simulink model "MSDR_v1.1"  (R2018a)
settings: Solver=ode3  StartTime=0.0  StopTime=21600  FixedStep=0.05
values from neighbouring files (symbols this model uses):
  a_f = -3.22E-5    (= -3.22e-05)    [MSDR_parameters.m]
  a_g = +2.35E-5    (= 2.35e-05)    [MSDR_parameters.m]
  A_s = 1.2245    [MSDR_parameters.m]
  beta = [0.000223, 0.001457, 0.001307, 0.002628, 0.000766, 0.000280]    [MSDR_parameters.m]
  beta_t = sum(beta)    [MSDR_parameters.m]
  ce1 = 1.2471e-07    [MSDR_parameters.m]
  ce2 = 5.3816e-14    [MSDR_parameters.m]
  ce3 = 3.3721e-08    [MSDR_parameters.m]
  Cp_fw = 3200.448e-6    (= 0.003200448)    [MSDR_parameters.m]
  Cp_hr = 0.0021520    (= 0.002152)    [MSDR_parameters.m]
  Cp_p = Cp_s_shx    (= 0.00154912)    [MSDR_parameters.m]
  Cp_s = Cp_s*1e-6    (= 3.588208e-09)    [MSDR_parameters.m]
  Cp_s_shx = 1549.12e-6    (= 0.00154912)    [MSDR_parameters.m]
  Cp_sc = 4761.392e-6    (= 0.004761392)    [MSDR_parameters.m]
  Cp_w = 456.056e-6    (= 0.000456056)    [MSDR_parameters.m]
  D_it = 0.0141478    [MSDR_parameters.m]
  D_ot = 0.015875    [MSDR_parameters.m]
  dHs_dPs = -0.042433622114357    (= -0.0424336221144)    [MSDR_parameters.m]
  eta_hp_isen = 0.861    [MSDR_parameters.m]
  eta_lp_isen = 0.861    [MSDR_parameters.m]
  gamma_I = 5.1135e-2    (= 0.051135)    [MSDR_parameters.m]
  gamma_Xe = 1.1628e-2    (= 0.011628)    [MSDR_parameters.m]
  H_fwh1 = 0.46009    [MSDR_parameters.m]
  h_fwh1 = 0.5927    [MSDR_parameters.m]
  H_fwh2 = 0.6784    [MSDR_parameters.m]
  h_fwh2 = 0.5927    [MSDR_parameters.m]
  H_lp_isen = 958.4*1054.35e-6/0.45359237    (= 2.22774699671)    [MSDR_parameters.m]
  H_nc = 3.2952    [MSDR_parameters.m]
  h_pw = h_s_shx    (= 0.00567446)    [MSDR_parameters.m]
  H_rh = 2.8115    [MSDR_parameters.m]
  h_wb = 13349.334646671E-6    (= 0.0133493346467)    [MSDR_parameters.m]
  h_ws = 5732.378387768E-6    (= 0.00573237838777)    [MSDR_parameters.m]
  h_wsc = 8385.005556375E-6    (= 0.00838500555638)    [MSDR_parameters.m]
  hA_fg = [h_fg*A_fg/2, h_fg*A_fg/2]    [MSDR_parameters.m]
  hA_p_phx1 = h_p_phx*A_p_phx    [MSDR_parameters.m]
  hA_p_phx2 = h_p_phx*A_p_phx    [MSDR_parameters.m]
  hA_p_phx3 = h_p_phx*A_p_phx    [MSDR_parameters.m]
  hA_p_phx4 = h_p_phx*A_p_phx    [MSDR_parameters.m]
  hA_p_phx5 = h_p_phx*A_p_phx    [MSDR_parameters.m]
  hA_p_phx6 = h_p_phx*A_p_phx    [MSDR_parameters.m]
  hA_p_shx1 = h_p_shx*A_p_shx    [MSDR_parameters.m]
  hA_p_shx2 = h_p_shx*A_p_shx    [MSDR_parameters.m]
  hA_p_shx3 = h_p_shx*A_p_shx    [MSDR_parameters.m]
  hA_p_shx4 = h_p_shx*A_p_shx    [MSDR_parameters.m]
  hA_p_shx5 = h_p_shx*A_p_shx    [MSDR_parameters.m]
  hA_p_shx6 = h_p_shx*A_p_shx    [MSDR_parameters.m]
  hA_s_phx1 = h_s_phx*A_s_phx    [MSDR_parameters.m]
  hA_s_phx2 = h_s_phx*A_s_phx    [MSDR_parameters.m]
  hA_s_phx3 = h_s_phx*A_s_phx    [MSDR_parameters.m]
  hA_s_phx4 = h_s_phx*A_s_phx    [MSDR_parameters.m]
  hA_s_phx5 = h_s_phx*A_s_phx    [MSDR_parameters.m]
  hA_s_phx6 = h_s_phx*A_s_phx    [MSDR_parameters.m]
  hA_s_shx1 = h_s_shx*A_s_shx    [MSDR_parameters.m]
  hA_s_shx2 = h_s_shx*A_s_shx    [MSDR_parameters.m]
  hA_s_shx3 = h_s_shx*A_s_shx    [MSDR_parameters.m]
  hA_s_shx4 = h_s_shx*A_s_shx    [MSDR_parameters.m]
  hA_s_shx5 = h_s_shx*A_s_shx    [MSDR_parameters.m]
  hA_s_shx6 = h_s_shx*A_s_shx    [MSDR_parameters.m]
  I_0 = gamma_I*Sig_f_msdr*phi_0/lam_I    (= 4.38204721773e+16)    [MSDR_parameters.m]
  Ifa = [0.25, 0.25]    [MSDR_parameters.m]
  Ifb = [0.25, 0.25]    [MSDR_parameters.m]
  Ig = [0.5, 0.5]    [MSDR_parameters.m]
  K_1 = 11.632248097704855    (= 11.6322480977)    [MSDR_parameters.m]
  K_4 = b(1)    [MSDR_parameters.m]
  K_5 = a(1)    [MSDR_parameters.m]
  K_b = 12.834854076292217    (= 12.8348540763)    [MSDR_parameters.m]
  K_b_hp = 0.1634    [MSDR_parameters.m]
  K_b_lp = 0.2174    [MSDR_parameters.m]
  K_sc = -17.615718797133468    (= -17.6157187971)    [MSDR_parameters.m]
  ka = [0.235, 0.235]    [MSDR_parameters.m]
  kb = [0.235, 0.235]    [MSDR_parameters.m]
  kga = [0.015, 0.015]    [MSDR_parameters.m]
  kgb = [0.015, 0.015]    [MSDR_parameters.m]
  L = 8.5344    [MSDR_parameters.m]
  L_b = 2.3645    [MSDR_parameters.m]
  L_s = 4.723    [MSDR_parameters.m]
  Lam = 2.400E-04    (= 0.00024)    [MSDR_parameters.m]
  lam = [0.0124, 0.0305, 0.111, 0.301, 1.14, 3.01]    [MSDR_parameters.m]
  lam_bubl = 2.0e-2    (= 0.02)    [MSDR_parameters.m]
  lam_I = 2.875e-5    (= 2.875e-05)    [MSDR_parameters.m]
  lam_Xe = 2.0916e-5    (= 2.0916e-05)    [MSDR_parameters.m]
  m_3m = W_3*2    (= 8618.207327)    [MSDR_parameters.m]
  m_fm = W_f*2    (= 9978.96)    [MSDR_parameters.m]
  m_sb = 1717    [MSDR_parameters.m]
  M_stm = 0.018    [MSDR_parameters.m]
  mb_cpb = 2.689619410657651e+00    (= 2.68961941066)    [MSDR_parameters.m]
  mcp_fa = mfa*Cp_f    [MSDR_parameters.m]
  mcp_fb = mfb*Cp_f    [MSDR_parameters.m]
  mcp_g = mg*Cp_g    [MSDR_parameters.m]
  mcp_p_phx1 = Cp_p_phx*mp_phx1    [MSDR_parameters.m]
  mcp_p_phx2 = Cp_p_phx*mp_phx2    [MSDR_parameters.m]
  mcp_p_phx3 = Cp_p_phx*mp_phx3    [MSDR_parameters.m]
  mcp_p_phx4 = Cp_p_phx*mp_phx4    [MSDR_parameters.m]
  mcp_p_phx5 = Cp_p_phx*mp_phx5    [MSDR_parameters.m]
  mcp_p_phx6 = Cp_p_phx*mp_phx6    [MSDR_parameters.m]
  mcp_p_shx1 = Cp_p_shx*mp_shx1    [MSDR_parameters.m]
  mcp_p_shx2 = Cp_p_shx*mp_shx2    [MSDR_parameters.m]
  mcp_p_shx3 = Cp_p_shx*mp_shx3    [MSDR_parameters.m]
  mcp_p_shx4 = Cp_p_shx*mp_shx4    [MSDR_parameters.m]
  mcp_p_shx5 = Cp_p_shx*mp_shx5    [MSDR_parameters.m]
  mcp_p_shx6 = Cp_p_shx*mp_shx6    [MSDR_parameters.m]
  mcp_s_phx1 = Cp_s_phx*ms_phx1    [MSDR_parameters.m]
  mcp_s_phx2 = Cp_s_phx*ms_phx2    [MSDR_parameters.m]
  mcp_s_phx3 = Cp_s_phx*ms_phx3    [MSDR_parameters.m]
  mcp_s_phx4 = Cp_s_phx*ms_phx4    [MSDR_parameters.m]
  mcp_s_phx5 = Cp_s_phx*ms_phx5    [MSDR_parameters.m]
  mcp_s_phx6 = Cp_s_phx*ms_phx6    [MSDR_parameters.m]
  mcp_s_shx1 = Cp_s_shx*ms_shx1    [MSDR_parameters.m]
  mcp_s_shx2 = Cp_s_shx*ms_shx1    [MSDR_parameters.m]
  mcp_s_shx3 = Cp_s_shx*ms_shx1    [MSDR_parameters.m]
  mcp_s_shx4 = Cp_s_shx*ms_shx1    [MSDR_parameters.m]
  mcp_s_shx5 = Cp_s_shx*ms_shx1    [MSDR_parameters.m]
  mcp_s_shx6 = Cp_s_shx*ms_shx1    [MSDR_parameters.m]
  mcp_t_phx1 = Cp_t_phx*mt_phx1    [MSDR_parameters.m]
  mcp_t_phx2 = Cp_t_phx*mt_phx2    [MSDR_parameters.m]
  mcp_t_phx3 = Cp_t_phx*mt_phx3    [MSDR_parameters.m]
  mcp_t_phx4 = Cp_t_phx*mt_phx4    [MSDR_parameters.m]
  mcp_t_phx5 = Cp_t_phx*mt_phx5    [MSDR_parameters.m]
  mcp_t_phx6 = Cp_t_phx*mt_phx6    [MSDR_parameters.m]
  mcp_t_shx1 = Cp_t_phx*mt_shx1    [MSDR_parameters.m]
  ... (+177 more)
undefined symbols (not defined in the file or in its folder): C0, H_rh_table, H_rh_table1, H_rh_table2, H_rhvap_table, H_s_table, H_table, hA_p_thx1, hA_p_thx2, hA_p_thx3, hA_s_thx1, hA_s_thx2, hA_s_thx3, mcp_p_thx1, mcp_p_thx2, mcp_p_thx3, mcp_s_thx1, mcp_s_thx2, mcp_s_thx3, mcp_t_thx1, mcp_t_thx2, mcp_t_thx3, mp_thx1, mp_thx2, mp_thx3, ms_thx1, ms_thx2, ms_thx3, P_nc_table, P_rh_table, P_rh_table1, pres_table, rho_rh_table, rho_table, SV_nc_table, T0_p_thx1, T0_p_thx2, T0_p_thx3, T0_s_thx1, T0_s_thx2, T0_s_thx3, T0_t_thx1, T0_t_thx2, T0_t_thx3, temp_table, u14, Wp_thx1, Wp_thx2
libraries: simulink x13
(part 3 of 6)

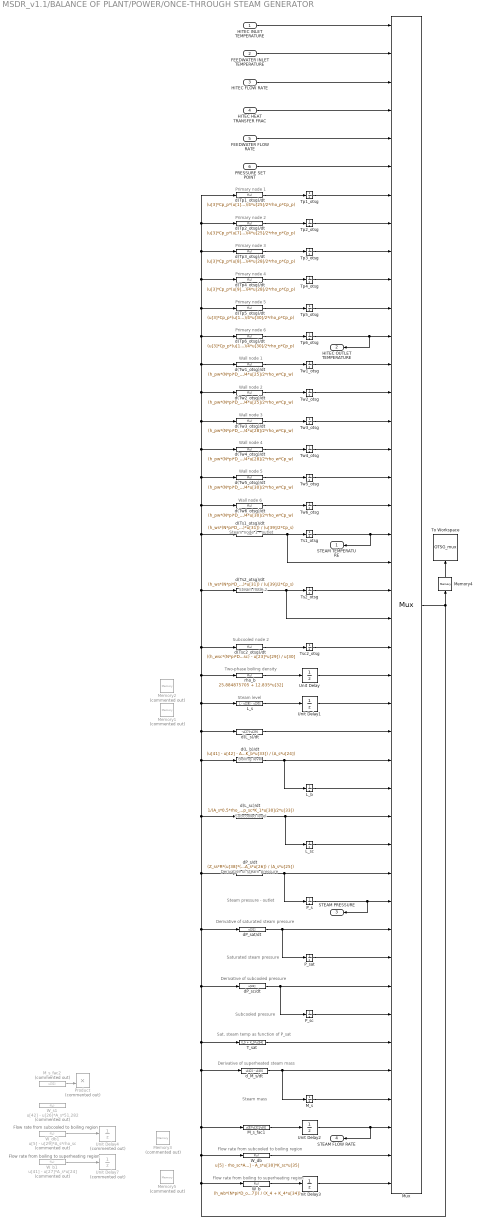
== system MSDR_v1.1/BALANCE OF PLANT/POWER/ONCE-THROUGH STEAM GENERATOR ==
  note: Primary node 1
  note: Primary node 2
  note: Primary node 3
  note: Primary node 4
  note: Primary node 5
  note: Primary node 6
  note: Wall node 1
  note: Wall node 2
  note: Wall node 3
  note: Wall node 4
  note: Wall node 5
  note: Wall node 6
  note: Steam node 1 - outlet
  note: Steam level
  note: Boiling level
  note: Subcooled level
  note: Derivative of saturated steam pressure
  note: Sat. steam temp as function of P_sat
  note: Saturated steam pressure
  note: Subcooled pressure
  note: Derivative of steam pressure
  note: Derivative of subcooled pressure
  note: Steam pressure - outlet
  note: Subcooled node 2
  note: Steam node 2
  note: Two-phase boiling density
  note: Derivative of superheated steam mass
  note: Steam mass
  note: Flow rate from subcooled to boiling region
  note: Flow rate from boiling to superheating region
  note: Flow rate from subcooled to boiling region
  note: Flow rate from boiling to superheating region
  HITEC INLET TEMPERATURE : Inport
  FEEDWATER INLET TEMPERATURE : Inport  Port=2
  HITEC FLOW RATE : Inport  Port=3
  HITEC HEAT TRANSFER FRAC : Inport  Port=4
  FEEDWATER FLOW RATE : Inport  Port=5
  PRESSURE SET POINT : Inport  Port=6
  L_b : Integrator  InitialCondition=L_b
  L_s : Fcn  Expr=L - u[28] - u[30]
  L_sc : Integrator  InitialCondition=.5344
  M_s : Integrator  InitialCondition=A_s*rho_s*L_s
  M_s_fac1 : Fcn  Expr=u[5]*u[32]/u[6]
  M_s_fac2 : Fcn  Commented=on  Expr=u[32]
  Memory1 : Memory  Commented=on  InitialCondition=L_s  InheritSampleTime=on
  Memory2 : Memory  Commented=on  InitialCondition=rho_b  InheritSampleTime=on
  Memory3 : Memory  Commented=on  InitialCondition=W_fw  InheritSampleTime=on
  Memory4 : Memory  InheritSampleTime=on
  Memory5 : Memory  Commented=on  InitialCondition=W_fw  InheritSampleTime=on
  Mux : Mux  Inputs=42
      settings: DisplayOption=signals
  P_s : Integrator  InitialCondition=P_s
  P_sat : Integrator  InitialCondition=P_sat
  P_sc : Integrator  InitialCondition=P_sc
  Product : Product  Commented=on
  T_sat : Fcn  Expr=X_5 + K_5*u[34]
  To Workspace : ToWorkspace  VariableName=OTSG_mux  SampleTime=-1
  Tp1_otsg : Integrator  InitialCondition=T_p1
  Tp2_otsg : Integrator  InitialCondition=T_p2
  Tp3_otsg : Integrator  InitialCondition=T_p3
  Tp4_otsg : Integrator  InitialCondition=T_p4
  Tp5_otsg : Integrator  InitialCondition=T_p5
  Tp6_otsg : Integrator  InitialCondition=T_p6
  Ts1_otsg : Integrator  InitialCondition=T_s1
  Ts2_otsg : Integrator  InitialCondition=T_s2
  Tsc2_otsg : Integrator  InitialCondition=T_sc2
  Tw1_otsg : Integrator  InitialCondition=T_w1
  Tw2_otsg : Integrator  InitialCondition=T_w2
  Tw3_otsg : Integrator  InitialCondition=T_w3
  Tw4_otsg : Integrator  InitialCondition=T_w4
  Tw5_otsg : Integrator  InitialCondition=T_w5
  Tw6_otsg : Integrator  InitialCondition=T_w6
  Unit Delay : UnitDelay  InitialCondition=rho_b  SampleTime=-1
  Unit Delay1 : UnitDelay  InitialCondition=L_s  SampleTime=-1
  Unit Delay2 : UnitDelay  InitialCondition=W_fw  SampleTime=-1
  Unit Delay3 : UnitDelay  InitialCondition=W_fw  SampleTime=-1
  Unit Delay4 : UnitDelay  Commented=on  InitialCondition=W_fw  SampleTime=-1
  Unit Delay7 : UnitDelay  Commented=on  InitialCondition=W_fw  SampleTime=-1
  W_b : Fcn  Expr=(h_wb*(N*pi*D_ot*u[28])*(0.5*u[15] + 0.5*u[16] - u[37])) / (X_4 + K_4*u[34])
  W_b1 : Fcn  Commented=on  Expr=u[41] - u[27]*A_s*u[24]
  W_db : Fcn  Expr=u[5] - rho_sc*A_s*u[29] - A_s*u[30]*K_sc*u[35]
  W_db1 : Fcn  Commented=on  Expr=u[5] - u[29]*A_s*rho_sc
  W_s1 : Fcn  Commented=on  Expr=u[42] - u[26]*A_s*51.282
  d(L_b)/dt : Fcn  Expr=(u[41] - u[42] - A_s*u[28]*K_b*u[33]) / (A_s*u[24])
  d(L_s)/dt : Fcn  Expr=-u[27]-u[29]
  d(L_sc)/dt : Fcn  Expr=1/(A_s*0.5*rho_sc*Cp_sc*(u[23] - u[37])) * (h_wsc*N*pi*D_ot*u[30]/2*(u[17] - u[37]) + u[5]*Cp_sc*(u[23] - u[37]) - A_s*u[30]/2*(K_sc*Cp_sc*(u[23] - 2*u[37]) - 1)*u[35] - A_s*rho_sc*Cp_sc*K_1*u[30]/2*u[33])
  d(Tp1_otsg)/dt : Fcn  Expr=(u[3]*Cp_p*(u[1] - u[7]) + h_pw*(N*pi*D_it*u[25]/2)*(u[13] - u[7])) / (N*pi*(D_it^2)/4*u[25]/2*rho_p*Cp_p)
  d(Tp2_otsg)/dt : Fcn  Expr=(u[3]*Cp_p*(u[7] - u[8]) + h_pw*(N*pi*D_it*u[25]/2)*(u[14] - u[8])) / (N*pi*(D_it^2)/4*u[25]/2*rho_p*Cp_p)
  d(Tp3_otsg)/dt : Fcn  Expr=(u[3]*Cp_p*(u[8] - u[9]) + h_pw*(N*pi*D_it*u[28]/2)*(u[15] - u[9])) / (N*pi*(D_it^2)/4*u[28]/2*rho_p*Cp_p)
  d(Tp4_otsg)/dt : Fcn  Expr=(u[3]*Cp_p*(u[9] - u[10]) + h_pw*(N*pi*D_it*u[28]/2)*(u[16] - u[10])) / (N*pi*(D_it^2)/4*u[28]/2*rho_p*Cp_p)
  d(Tp5_otsg)/dt : Fcn  Expr=(u[3]*Cp_p*(u[10] - u[11]) + h_pw*(N*pi*D_it*u[30]/2)*(u[17] - u[11])) / (N*pi*(D_it^2)/4*u[30]/2*rho_p*Cp_p)
  d(Tp6_otsg)/dt : Fcn  Expr=(u[3]*Cp_p*(u[11] - u[12]) + h_pw*(N*pi*D_it*u[30]/2)*(u[18] - u[12])) / (N*pi*(D_it^2)/4*u[30]/2*rho_p*Cp_p)
  d(Ts1_otsg)/dt : Fcn  Expr=(h_ws*(N*pi*D_ot*u[25]/2)*(u[13] - u[19]) + u[40]*Cp_s*(u[21] - u[19]) + Cp_s*(u[21] - u[19])*u[38]/2 + (A_s*u[25]/2 - u[39]/2*dHs_dPs)*u[31]) / (u[39]/2*Cp_s)
  d(Ts2_otsg)/dt : Fcn  Expr=(h_ws*(N*pi*D_ot*u[25]/2)*(u[14] - u[21]) + u[42]*Cp_s*(u[37] - u[21]) + (A_s*u[25]/2 - u[39]/2*dHs_dPs)*u[31]) / (u[39]/2*Cp_s)
  d(Tsc2_otsg)/dt : Fcn  Expr=((h_wsc*(N*pi*D_ot*u[30]/2)*(u[18] - u[23]) + Cp_sc*(u[5]*u[2] - (u[5] + u[41])*0.5*u[23]) + A_s*u[30]/2*u[35]) * 2/(A_s*rho_sc*Cp_sc) - u[23]*u[29]) / u[30]
  d(Tw1_otsg)/dt : Fcn  Expr=(h_pw*(N*pi*D_it*u[25]/2)*(u[7] - u[13]) + h_ws*(N*pi*D_ot*u[25]/2)*(u[19] - u[13])) / (N*pi*(D_ot^2 - D_it^2)/4*u[25]/2*rho_w*Cp_w)
  d(Tw2_otsg)/dt : Fcn  Expr=(h_pw*(N*pi*D_it*u[25]/2)*(u[8] - u[14]) + h_ws*(N*pi*D_ot*u[25]/2)*(u[21] - u[14])) / (N*pi*(D_ot^2 - D_it^2)/4*u[25]/2*rho_w*Cp_w)
  d(Tw3_otsg)/dt : Fcn  Expr=(h_pw*(N*pi*D_it*u[28]/2)*(u[9] - u[15]) + h_wb*(N*pi*D_ot*u[28]/2)*(u[37] - u[15])) / (N*pi*(D_ot^2 - D_it^2)/4*u[28]/2*rho_w*Cp_w)
  d(Tw4_otsg)/dt : Fcn  Expr=(h_pw*(N*pi*D_it*u[28]/2)*(u[10] - u[16]) + h_wb*(N*pi*D_ot*u[28]/2)*(u[37] - u[16])) / (N*pi*(D_ot^2 - D_it^2)/4*u[28]/2*rho_w*Cp_w)
  d(Tw5_otsg)/dt : Fcn  Expr=(h_pw*(N*pi*D_it*u[30]/2)*(u[11] - u[17]) + h_wsc*(N*pi*D_ot*u[30]/2)*(u[37] - u[17])) / (N*pi*(D_ot^2 - D_it^2)/4*u[30]/2*rho_w*Cp_w)
  d(Tw6_otsg)/dt : Fcn  Expr=(h_pw*(N*pi*D_it*u[30]/2)*(u[12] - u[18]) + h_wsc*(N*pi*D_ot*u[30]/2)*(u[23] - u[18])) / (N*pi*(D_ot^2 - D_it^2)/4*u[30]/2*rho_w*Cp_w)
  dP_s/dt : Fcn  Expr=(Z_ss*R*(u[38]*(u[19] + u[21]) + u[39]*(u[20] + u[22]))/(2*M_stm) - u[32]*A_s*u[26]) / (A_s*u[25])
  dP_sat/dt : Fcn  Expr=u[31]
  dP_sc/dt : Fcn  Expr=u[31]
  d_M_s/dt : Fcn  Expr=u[42] - u[40]
  rho_b : Fcn  Expr=25.884875705 + 12.835*u[32]
  STEAM TEMPERATURE : Outport
  HITEC OUTLET TEMPERATURE : Outport  Port=2
  STEAM PRESSURE : Outport  Port=3
  STEAM FLOW RATE : Outport  Port=4
  wires:
  FEEDWATER INLET TEMPERATURE/1 -> Mux/2
  d(Tp1_otsg)/dt/1 -> Tp1_otsg/1
  HITEC INLET TEMPERATURE/1 -> Mux/1
  HITEC FLOW RATE/1 -> Mux/3
  HITEC HEAT TRANSFER FRAC/1 -> Mux/4
  FEEDWATER FLOW RATE/1 -> Mux/5
  PRESSURE SET POINT/1 -> Mux/6
  Tp1_otsg/1 -> Mux/7
  Tp2_otsg/1 -> Mux/8
  d(Tp2_otsg)/dt/1 -> Tp2_otsg/1
  Tp3_otsg/1 -> Mux/9
  d(Tp3_otsg)/dt/1 -> Tp3_otsg/1
  Tp4_otsg/1 -> Mux/10
  d(Tp4_otsg)/dt/1 -> Tp4_otsg/1
  Tp5_otsg/1 -> Mux/11
  d(Tp5_otsg)/dt/1 -> Tp5_otsg/1
  d(Tp6_otsg)/dt/1 -> Tp6_otsg/1
  Tp6_otsg/1 -> HITEC OUTLET TEMPERATURE/1, Mux/12
  Tw1_otsg/1 -> Mux/13
  d(Tw1_otsg)/dt/1 -> Tw1_otsg/1
  d(Tw2_otsg)/dt/1 -> Tw2_otsg/1
  Tw2_otsg/1 -> Mux/14
  Tw3_otsg/1 -> Mux/15
  d(Tw3_otsg)/dt/1 -> Tw3_otsg/1
  d(Tw4_otsg)/dt/1 -> Tw4_otsg/1
  Tw4_otsg/1 -> Mux/16
  Tw5_otsg/1 -> Mux/17
  d(Tw5_otsg)/dt/1 -> Tw5_otsg/1
  d(Tw6_otsg)/dt/1 -> Tw6_otsg/1
  Tw6_otsg/1 -> Mux/18
  Ts1_otsg/1 -> STEAM TEMPERATURE/1, Mux/19
  L_sc/1 -> Mux/30
  L_s/1 -> Unit Delay1/1
  L_b/1 -> Mux/28
  P_s/1 -> Mux/32, STEAM PRESSURE/1
  P_sat/1 -> Mux/34
  P_sc/1 -> Mux/36
  Tsc2_otsg/1 -> Mux/23
  d(Tsc2_otsg)/dt/1 -> Tsc2_otsg/1
  Ts2_otsg/1 -> Mux/21
  rho_b/1 -> Unit Delay/1
  Unit Delay/1 -> Mux/24
  M_s/1 -> Mux/39
  Memory4/1 -> To Workspace/1
  Mux/1 -> Memory4/1, W_b/1, W_db/1, d_M_s/dt/1, T_sat/1, dP_sc/dt/1, dP_sat/dt/1, dP_s/dt/1, d(L_sc)/dt/1, d(L_b)/dt/1, d(L_s)/dt/1, L_s/1, rho_b/1, d(Tsc2_otsg)/dt/1, d(Ts2_otsg)/dt/1, d(Ts1_otsg)/dt/1, d(Tw6_otsg)/dt/1, d(Tw5_otsg)/dt/1, d(Tw4_otsg)/dt/1, d(Tw3_otsg)/dt/1, d(Tw2_otsg)/dt/1, d(Tw1_otsg)/dt/1, d(Tp6_otsg)/dt/1, d(Tp5_otsg)/dt/1, d(Tp4_otsg)/dt/1, d(Tp3_otsg)/dt/1, d(Tp2_otsg)/dt/1, d(Tp1_otsg)/dt/1, M_s_fac1/1
  W_b1/1 -> Unit Delay7/1
  W_db1/1 -> Unit Delay4/1
  M_s_fac2/1 -> Product/2
  d(Ts1_otsg)/dt/1 -> Mux/20, Ts1_otsg/1
  d(Ts2_otsg)/dt/1 -> Mux/22, Ts2_otsg/1
  dP_s/dt/1 -> Mux/31, P_s/1
  d(L_b)/dt/1 -> Mux/27, L_b/1
  d(L_s)/dt/1 -> Mux/26
  d(L_sc)/dt/1 -> Mux/29, L_sc/1
  dP_sat/dt/1 -> Mux/33, P_sat/1
  dP_sc/dt/1 -> Mux/35, P_sc/1
  Unit Delay1/1 -> Mux/25
  T_sat/1 -> Mux/37
  W_b/1 -> Unit Delay3/1
  M_s_fac1/1 -> Unit Delay2/1
  Unit Delay3/1 -> Mux/42
  d_M_s/dt/1 -> Mux/38, M_s/1
  W_db/1 -> Mux/41
  Unit Delay2/1 -> STEAM FLOW RATE/1, Mux/40

== system MSDR_v1.1/BALANCE OF PLANT/POWER/REHEATER ==
  note: Density of steam in reheater
  note: Enthalpy of steam in reheater
  note: Steam flow from reheater to LP turbine
  note: Enthalpy of saturated vapor as a function of reheater pressure
  note: Flow from reheater to feedwater heater 2
  note: Heat transfer rate in the reheater
  note: Temperature of shell side steam in reheater
  note: # keeping same density, doubled volume
  note: #doubled volume means double residence time
  note: #doubled volume means double residence time
  STEAM FLOW RATE - SECONDARY VALVE : Inport
  FLOW from MOISTURE SEPARATOR : Inport  Port=2
  STEAM TEMPERATURE : Inport  Port=3
  H_g : Fcn  Expr=u[7]
  H_rh : Integrator  InitialCondition=H_rh
  Mux : Mux  Inputs=12
      settings: DisplayOption=signals
  Q_rh : Integrator  InitialCondition=Q_rh
  RH H_liq : Lookup_n-D  NumberOfTableDimensions=1  BreakpointsForDimension1=P_rh_table1  Table=H_rh_table1  InternalRulePriority=Speed  RndMeth=Simplest  InputSameDT=on
  RH Pressure : Lookup_n-D  BreakpointsForDimension1=H_rh_table2  BreakpointsForDimension2=rho_rh_table  Table=P_rh_table  InternalRulePriority=Speed  RndMeth=Simplest  InputSameDT=on
  RH density : Fcn  Expr=u[5]
  RH enthalpy : Fcn  Expr=u[6]
  T_rh : Fcn  Expr=u[7]*M_stm/(u[5]*R)
  To Workspace : ToWorkspace  VariableName=RH_mux  SampleTime=0.1
      settings: Save2DSignal=2-D array (concatenate along first dimension)
  Unit Delay1 : UnitDelay  InitialCondition=203.11  SampleTime=-1
  Unit Delay2 : UnitDelay  InitialCondition=2.8029  SampleTime=-1
  Unit Delay3 : UnitDelay  InitialCondition=466.87  SampleTime=-1
  Unit Delay7 : UnitDelay  InitialCondition=2.8582  SampleTime=-1
  d(H_rh)/dt : Fcn  Expr=(u[11] + u[2]*u[9] - u[8]*u[6])/(u[5]*V_rh) + u[7]*(u[2] - u[8])/(u[5]^2*V_rh)
  d(Q_rh)/dt : Fcn  Expr=((u[1] + u[10])*Cp_hr*(u[3] - u[12]))/(2*tau_rhh) - u[11]/(tau_rhh)
  d(rho_rh)/dt : Fcn  Expr=(u[2] - u[8])/(V_rh)
  d(w'_rh_fwh2)/dt : Fcn  Expr=(u[1] - u[10])/(tau_rh1)
  rho_rh : Integrator  InitialCondition=rho_rh
  w'_rh_fwh2 : Integrator  InitialCondition=51.447
  w_3 : Fcn  Expr=33*(u[7]*u[5])^0.5
  "FLOW to LP TURBINE " : Outport
  FLOW to FWH2 : Outport  Port=2
  STEAM PRESSURE - REHEATER : Outport  Port=3
  STEAM ENTHALPY - REHEATER : Outport  Port=4
  wires:
  STEAM FLOW RATE - SECONDARY VALVE/1 -> Mux/1
  FLOW from MOISTURE SEPARATOR/1 -> Mux/2
  STEAM TEMPERATURE/1 -> Mux/3
  H_rh/1 -> STEAM ENTHALPY - REHEATER/1, Mux/6
  d(H_rh)/dt/1 -> H_rh/1
  rho_rh/1 -> Mux/5
  d(rho_rh)/dt/1 -> rho_rh/1, Mux/4
  Unit Delay7/1 -> Mux/7, STEAM PRESSURE - REHEATER/1
  RH density/1 -> RH Pressure/2
  RH Pressure/1 -> Unit Delay7/1
  RH enthalpy/1 -> RH Pressure/1
  Unit Delay1/1 -> "FLOW to LP TURBINE "/1, Mux/8
  w_3/1 -> Unit Delay1/1
  H_g/1 -> RH H_liq/1
  Unit Delay2/1 -> Mux/9
  d(w'_rh_fwh2)/dt/1 -> w'_rh_fwh2/1
  w'_rh_fwh2/1 -> FLOW to FWH2/1, Mux/10
  d(Q_rh)/dt/1 -> Q_rh/1
  Q_rh/1 -> Mux/11
  T_rh/1 -> Unit Delay3/1
  Mux/1 -> To Workspace/1, T_rh/1, d(Q_rh)/dt/1, d(w'_rh_fwh2)/dt/1, H_g/1, w_3/1, RH enthalpy/1, d(H_rh)/dt/1, d(rho_rh)/dt/1, RH density/1
  RH H_liq/1 -> Unit Delay2/1
  Unit Delay3/1 -> Mux/12

== system MSDR_v1.1/BALANCE OF PLANT/POWER/SECONDARY STEAM VALVE ==
  STEAM FROM OTSG : Inport
  Product : Product
  SSV Coefficient 16% diverted to reheater : Constant  Value=.16
  STEAM TO REHEATER : Outport
  wires:
  STEAM FROM OTSG/1 -> Product/2
  Product/1 -> STEAM TO REHEATER/1
  SSV Coefficient 16% diverted to reheater/1 -> Product/1

== system MSDR_v1.1/HEAT EXCHANGERS/HEAT EXCHANGER LOOP 1/BOILER & REHEATER ==
  Coolant Inlet Temp : Inport
  Power Demand (Frac) : Inport  Port=2
  Fcn : Fcn  Commented=on  Expr=u[1] - u[2]*250/((Ws_shx1 + Ws_shx2)*Cp_s_shx)
  Integrator : Integrator  InitialCondition=400
  Mux : Mux  Inputs=3
      settings: DisplayOption=signals
  To Workspace : ToWorkspace  VariableName=msdr_br_mux1  SampleTime=-1
  ddt_t_b = 1/tau_b*(t_bin-t_b)-p_b/mb_cpb : Fcn  Expr=W_sb*(u(1)-u(3))/m_sb - u(2)/mb_cpb
  Coolant Exit Temp : Outport
  wires:
  Mux/1 -> ddt_t_b = 1/tau_b*(t_bin-t_b)-p_b/mb_cpb/1, To Workspace/1
  Power Demand (Frac)/1 -> Mux/2
  Coolant Inlet Temp/1 -> Mux/1
  ddt_t_b = 1/tau_b*(t_bin-t_b)-p_b/mb_cpb/1 -> Integrator/1
  Integrator/1 -> Coolant Exit Temp/1, Mux/3

== system MSDR_v1.1/HEAT EXCHANGERS/HEAT EXCHANGER LOOP 1/Fractional Power Demand (fractional) ==
  Add : Sum
  Constant : Constant
  Saturation : Saturate  UpperLimit=1  LowerLimit=0.2
  Saturation1 : Saturate  UpperLimit=.8  LowerLimit=0
  Slider : Subsystem  DialogController=hmiCreateDDGDialog  IsWebBlock=on  mask(MWDashboardBlock){webBlockId=20dd6961-4cd4-422a-ae50-f434dac2eac1, webBlockType=slider, ShowInLibBrowser=on, ShowInitialText=on, HMISrcModelName=OTSG_v1_1}
      mask prompts: webBlockId "WebBlock Id"; webBlockType "WebBlock Type"; HMISrcModelName "Source Model"
      mask help: SimulinkHMI:dialogs:SliderDialogDesc
      mask Help: helpview([docroot '/mapfiles/simulink.map'], 'hmi_slider')
      mask Display:
      | if strcmp(get_param(bdroot(gcb),'BlockDiagramType'), 'library')
      |     image([(matlabroot) '/toolbox/simulink/hmi/icons/Slider.png']);
      | end
  down 1%/min : simulink/Sources/Ramp  slope=-0.01/60  start=2500  InitialOutput=1
  up 1%/min1 : simulink/Sources/Ramp  slope=0.01/60  start=2500+3600+5000  InitialOutput=0
  Power Demand(frac) : Outport
  wires:
  down 1%/min/1 -> Saturation/1
  Saturation/1 -> Add/1
  up 1%/min1/1 -> Saturation1/1
  Saturation1/1 -> Add/2
  Constant/1 -> Power Demand(frac)/1

== system MSDR_v1.1/HEAT EXCHANGERS/HEAT EXCHANGER LOOP 1/PHX PRIM MIXING ==
  Tp_phx1 : Inport
  Tp_phx2 : Inport  Port=2
  p_flow_frac : Inport  Port=3
  Fcn : Fcn  Expr=u[3]*Wp_phx1/mp_phxm*(u[1]-u[4]) + u[3]*Wp_phx2/mp_phxm*(u[2]-u[4])
  Integrator : Integrator  InitialCondition=Tf_in
  Mux : Mux
  Tp_phx_mix : Outport
  wires:
  Tp_phx1/1 -> Mux/1
  Tp_phx2/1 -> Mux/2
  Mux/1 -> Fcn/1
  p_flow_frac/1 -> Mux/3
  Fcn/1 -> Integrator/1
  Integrator/1 -> Tp_phx_mix/1, Mux/4

== system MSDR_v1.1/HEAT EXCHANGERS/HEAT EXCHANGER LOOP 1/PHX SEC MIXING ==
  Ts_phx1 : Inport
  Ts_phx2 : Inport  Port=2
  s_flow_frac : Inport  Port=3
  Fcn : Fcn  Expr=u[3]*Ws_phx1/ms_phxm*(u[1]-u[4]) + u[3]*Ws_phx2/ms_phxm*(u[2]-u[4])
  Integrator : Integrator  InitialCondition=T0_s_phx1(4)
  Mux : Mux
  Ts_phx_mix : Outport
  wires:
  Ts_phx1/1 -> Mux/1
  Ts_phx2/1 -> Mux/2
  Mux/1 -> Fcn/1
  s_flow_frac/1 -> Mux/3
  Fcn/1 -> Integrator/1
  Integrator/1 -> Ts_phx_mix/1, Mux/4

== system MSDR_v1.1/HEAT EXCHANGERS/HEAT EXCHANGER LOOP 1/PHX//SHX PUMP ==
  1-D Lookup Table : Lookup_n-D  NumberOfTableDimensions=1  BreakpointsForDimension1=xdat  Table=ydat  InternalRulePriority=Speed  RndMeth=Simplest  InputSameDT=on
  Clock : Clock
  Fcn : Fcn  Expr=exp((1/tau_p)*u)
  Final convection flow rate : Constant  Value=therm_conv
  Scope : Scope
  Subtract : Sum  Inputs=-+
  Switch : Switch  Criteria=u2 > Threshold
  Transport Delay : TransportDelay  DelayTime=2000000000  InitialOutput=1
  FLOW FRACTION : Outport
  HEAT TRANSFER FRACTION : Outport  Port=2
  wires:
  Transport Delay/1 -> 1-D Lookup Table/1, Scope/1, FLOW FRACTION/1
  Clock/1 -> Fcn/1
  Switch/1 -> Transport Delay/1
  Fcn/1 -> Subtract/1, Switch/1
  Final convection flow rate/1 -> Subtract/2, Switch/3
  Subtract/1 -> Switch/2
  1-D Lookup Table/1 -> HEAT TRANSFER FRACTION/1

== system MSDR_v1.1/HEAT EXCHANGERS/HEAT EXCHANGER LOOP 1/PHX1 HEAT TRANSFER ==
  PRIMARY FLUID INLET TEMPERATURE : Inport
  SECONDARY FLUID INLET TEMPERATURE : Inport  Port=2
  PRIMARY FLOW FRACTION : Inport  Port=3
  PRIMARY HEAT TRANSFER FRACTION : Inport  Port=4
  SECONDARY FLOW FRACTION : Inport  Port=5
  SECONDARY HEAT TRANSFER FRACTION : Inport  Port=6
  Mux : Mux  Inputs=16
      settings: DisplayOption=signals
  To Workspace : ToWorkspace  VariableName=phx1_ht  SampleTime=-1
  Tp1_phx1 : Integrator  InitialCondition=T0_p_phx1(1)
  Tp2_phx1 : Integrator  InitialCondition=T0_p_phx1(2)
  "Tp3_phx1 " : Integrator  InitialCondition=T0_p_phx1(3)
  Tp4_phx1 : Integrator  InitialCondition=T0_p_phx1(4)
  Ts1_phx1 : Integrator  InitialCondition=T0_s_phx1(1)
  Ts2_phx1 : Integrator  InitialCondition=T0_s_phx1(2)
  Ts3_phx1 : Integrator  InitialCondition=T0_s_phx1(3)
  Ts4_phx1 : Integrator  InitialCondition=T0_s_phx1(4)
  Tt1_phx1 : Integrator  InitialCondition=T0_t_phx1(1)
  Tt2_phx1 : Integrator  InitialCondition=T0_t_phx1(2)
  d(Tp1_phx1)/dt : Fcn  Expr=(u[13]*Wp_phx1/mp_phx1(1))*(u[1] - u[3]) + (u[14]*hA_p_phx1(1)/mcp_p_phx1(1))*(u[7] - u[3])
  d(Tp2_phx1)/dt : Fcn  Expr=(u[13]*Wp_phx1/mp_phx1(2))*(u[3] - u[4]) + (u[14]*hA_p_phx1(2)/mcp_p_phx1(2))*(u[7] - u[3])
  d(Tp3_phx1)/dt : Fcn  Expr=(u[13]*Wp_phx1/mp_phx1(3))*(u[4] - u[5]) + (u[14]*hA_p_phx1(3)/mcp_p_phx1(3))*(u[8] - u[5])
  d(Tp4_phx1)/dt : Fcn  Expr=(u[13]*Wp_phx1/mp_phx1(4))*(u[5] - u[6]) + (u[14]*hA_p_phx1(4)/mcp_p_phx1(4))*(u[8] - u[5])
  d(Ts1_phx1)/dt : Fcn  Expr=(u[15]*Ws_phx1/ms_phx1(1))*(u[2] - u[9]) + (u[16]*hA_s_phx1(1)/mcp_s_phx1(1))*(u[8] - u[9])
  d(Ts2_phx1)/dt : Fcn  Expr=(u[15]*Ws_phx1/ms_phx1(2))*(u[9] - u[10]) + (u[16]*hA_s_phx1(2)/mcp_s_phx1(2))*(u[8] - u[9])
  d(Ts3_phx1)/dt : Fcn  Expr=(u[15]*Ws_phx1/ms_phx1(3))*(u[10] - u[11]) + (u[16]*hA_s_phx1(3)/mcp_s_phx1(3))*(u[7] - u[11])
  d(Ts4_phx1)/dt : Fcn  Expr=(u[15]*Ws_phx1/ms_phx1(4))*(u[11] - u[12]) + (u[16]*hA_s_phx1(4)/mcp_s_phx1(4))*(u[7] - u[11])
  d(Tt1_phx1)/dt : Fcn  Expr=(u[14]*(hA_p_phx1(1) + hA_p_phx1(2))/mcp_t_phx1(1))*(u[3] - u[7]) + (u[16]*(hA_s_phx1(1) + hA_s_phx1(2))/mcp_t_phx1(1))*(u[11] - u[7])
  d(Tt2_phx1)/dt : Fcn  Expr=(u[14]*(hA_p_phx1(3) + hA_p_phx1(4))/mcp_t_phx1(2))*(u[5] - u[8]) + (u[16]*(hA_s_phx1(3) + hA_s_phx1(4))/mcp_t_phx1(2))*(u[9] - u[8])
  PHX1 TEMPERATURES : Outport
  wires:
  Ts1_phx1/1 -> Mux/9
  Ts2_phx1/1 -> Mux/10
  d(Ts2_phx1)/dt/1 -> Ts2_phx1/1
  d(Tp4_phx1)/dt/1 -> Tp4_phx1/1
  Tt1_phx1/1 -> Mux/7
  d(Tp2_phx1)/dt/1 -> Tp2_phx1/1
  Tp4_phx1/1 -> Mux/6
  d(Tt2_phx1)/dt/1 -> Tt2_phx1/1
  SECONDARY FLUID INLET TEMPERATURE/1 -> Mux/2
  Tt2_phx1/1 -> Mux/8
  Mux/1 -> PHX1 TEMPERATURES/1, To Workspace/1, d(Ts4_phx1)/dt/1, d(Ts3_phx1)/dt/1, d(Ts1_phx1)/dt/1, d(Tt2_phx1)/dt/1, d(Tt1_phx1)/dt/1, d(Tp4_phx1)/dt/1, d(Tp3_phx1)/dt/1, d(Tp2_phx1)/dt/1, d(Tp1_phx1)/dt/1, d(Ts2_phx1)/dt/1
  d(Tp1_phx1)/dt/1 -> Tp1_phx1/1
  d(Ts4_phx1)/dt/1 -> Ts4_phx1/1
  Tp1_phx1/1 -> Mux/3
  d(Ts1_phx1)/dt/1 -> Ts1_phx1/1
  d(Ts3_phx1)/dt/1 -> Ts3_phx1/1
  Ts3_phx1/1 -> Mux/11
  Ts4_phx1/1 -> Mux/12
  "Tp3_phx1 "/1 -> Mux/5
  d(Tp3_phx1)/dt/1 -> "Tp3_phx1 "/1
  Tp2_phx1/1 -> Mux/4
  d(Tt1_phx1)/dt/1 -> Tt1_phx1/1
  PRIMARY FLUID INLET TEMPERATURE/1 -> Mux/1
  PRIMARY FLOW FRACTION/1 -> Mux/13
  PRIMARY HEAT TRANSFER FRACTION/1 -> Mux/14
  SECONDARY HEAT TRANSFER FRACTION/1 -> Mux/16
  SECONDARY FLOW FRACTION/1 -> Mux/15

== system MSDR_v1.1/HEAT EXCHANGERS/HEAT EXCHANGER LOOP 1/PHX1 MATERIAL TRANSPORT ==
  PHX1 TEMPERATURES : Inport
  wires:
  PHX1 TEMPERATURES/1 -> ?

== system MSDR_v1.1/HEAT EXCHANGERS/HEAT EXCHANGER LOOP 1/PHX2 HEAT TRANSFER ==
  PRIMARY FLUID INLET TEMPERATURE : Inport
  SECONDARY FLUID INLET TEMPERATURE : Inport  Port=2
  PRIMARY FLOW FRACTION : Inport  Port=3
  PRIMARY HEAT TRANSFER FRACTION : Inport  Port=4
  SECONDARY FLOW FRACTION : Inport  Port=5
  SECONDARY HEAT TRANSFER FRACTION : Inport  Port=6
  Mux : Mux  Inputs=16
      settings: DisplayOption=signals
  To Workspace : ToWorkspace  VariableName=phx2_ht  SampleTime=-1
  Tp1_phx2 : Integrator  InitialCondition=T0_p_phx2(1)
  Tp2_phx2 : Integrator  InitialCondition=T0_p_phx1(2)
  "Tp3_phx2 " : Integrator  InitialCondition=T0_p_phx2(3)
  Tp4_phx2 : Integrator  InitialCondition=T0_p_phx2(4)
  Ts1_phx2 : Integrator  InitialCondition=T0_s_phx2(1)
  Ts2_phx2 : Integrator  InitialCondition=T0_s_phx2(2)
  Ts3_phx2 : Integrator  InitialCondition=T0_s_phx2(3)
  Ts4_phx2 : Integrator  InitialCondition=T0_s_phx2(4)
  Tt1_phx2 : Integrator  InitialCondition=T0_t_phx2(1)
  Tt2_phx2 : Integrator  InitialCondition=T0_t_phx2(2)
  d(Tp1_phx2)/dt : Fcn  Expr=(u[13]*Wp_phx2/mp_phx2(1))*(u[1] - u[3]) + (u[14]*hA_p_phx2(1)/mcp_p_phx2(1))*(u[7] - u[3])
  d(Tp2_phx2)/dt : Fcn  Expr=(u[13]*Wp_phx2/mp_phx2(2))*(u[3] - u[4]) + (u[14]*hA_p_phx2(2)/mcp_p_phx2(2))*(u[7] - u[3])
  d(Tp3_phx2)/dt : Fcn  Expr=(u[13]*Wp_phx2/mp_phx2(3))*(u[4] - u[5]) + (u[14]*hA_p_phx2(3)/mcp_p_phx2(3))*(u[8] - u[5])
  d(Tp4_phx2)/dt : Fcn  Expr=(u[13]*Wp_phx2/mp_phx2(4))*(u[5] - u[6]) + (u[14]*hA_p_phx2(4)/mcp_p_phx2(4))*(u[8] - u[5])
  d(Ts1_phx2)/dt : Fcn  Expr=(u[15]*Ws_phx2/ms_phx2(1))*(u[2] - u[9]) + (u[16]*hA_s_phx2(1)/mcp_s_phx2(1))*(u[8] - u[9])
  d(Ts2_phx2)/dt : Fcn  Expr=(u[15]*Ws_phx2/ms_phx2(2))*(u[9] - u[10]) + (u[16]*hA_s_phx2(2)/mcp_s_phx2(2))*(u[8] - u[9])
  d(Ts3_phx2)/dt : Fcn  Expr=(u[15]*Ws_phx2/ms_phx2(3))*(u[10] - u[11]) + (u[16]*hA_s_phx2(3)/mcp_s_phx2(3))*(u[7] - u[11])
  d(Ts4_phx2)/dt : Fcn  Expr=(u[15]*Ws_phx2/ms_phx2(4))*(u[11] - u[12]) + (u[16]*hA_s_phx2(4)/mcp_s_phx2(4))*(u[7] - u[11])
  d(Tt1_phx2)/dt : Fcn  Expr=(u[14]*(hA_p_phx2(1) + hA_p_phx2(2))/mcp_t_phx2(1))*(u[3] - u[7]) + (u[16]*(hA_s_phx2(1) + hA_s_phx2(2))/mcp_t_phx2(1))*(u[11] - u[7])
  d(Tt2_phx2)/dt : Fcn  Expr=(u[14]*(hA_p_phx2(3) + hA_p_phx2(4))/mcp_t_phx2(2))*(u[5] - u[8]) + (u[16]*(hA_s_phx2(3) + hA_s_phx2(4))/mcp_t_phx2(2))*(u[9] - u[8])
  PHX2 TEMPERATURES : Outport
  wires:
  Ts1_phx2/1 -> Mux/9
  Ts2_phx2/1 -> Mux/10
  d(Ts2_phx2)/dt/1 -> Ts2_phx2/1
  d(Tp4_phx2)/dt/1 -> Tp4_phx2/1
  Tt1_phx2/1 -> Mux/7
  d(Tp2_phx2)/dt/1 -> Tp2_phx2/1
  Tp4_phx2/1 -> Mux/6
  d(Tt2_phx2)/dt/1 -> Tt2_phx2/1
  SECONDARY FLUID INLET TEMPERATURE/1 -> Mux/2
  Tt2_phx2/1 -> Mux/8
  Mux/1 -> To Workspace/1, PHX2 TEMPERATURES/1, d(Ts4_phx2)/dt/1, d(Ts3_phx2)/dt/1, d(Ts1_phx2)/dt/1, d(Tt2_phx2)/dt/1, d(Tt1_phx2)/dt/1, d(Tp4_phx2)/dt/1, d(Tp3_phx2)/dt/1, d(Tp2_phx2)/dt/1, d(Tp1_phx2)/dt/1, d(Ts2_phx2)/dt/1
  d(Tp1_phx2)/dt/1 -> Tp1_phx2/1
  d(Ts4_phx2)/dt/1 -> Ts4_phx2/1
  Tp1_phx2/1 -> Mux/3
  d(Ts1_phx2)/dt/1 -> Ts1_phx2/1
  d(Ts3_phx2)/dt/1 -> Ts3_phx2/1
  Ts3_phx2/1 -> Mux/11
  Ts4_phx2/1 -> Mux/12
  "Tp3_phx2 "/1 -> Mux/5
  d(Tp3_phx2)/dt/1 -> "Tp3_phx2 "/1
  Tp2_phx2/1 -> Mux/4
  d(Tt1_phx2)/dt/1 -> Tt1_phx2/1
  PRIMARY FLUID INLET TEMPERATURE/1 -> Mux/1
  PRIMARY FLOW FRACTION/1 -> Mux/13
  PRIMARY HEAT TRANSFER FRACTION/1 -> Mux/14
  SECONDARY FLOW FRACTION/1 -> Mux/15
  SECONDARY HEAT TRANSFER FRACTION/1 -> Mux/16

== system MSDR_v1.1/HEAT EXCHANGERS/HEAT EXCHANGER LOOP 1/PHX2 MATERIAL TRANSPORT ==
  PHX2 TEMPERATURES : Inport
  wires:
  PHX2 TEMPERATURES/1 -> ?

== system MSDR_v1.1/HEAT EXCHANGERS/HEAT EXCHANGER LOOP 1/SHX PRIM MIXING ==
  Tp_shx1 : Inport
  Tp_shx2 : Inport  Port=2
  p_flow_frac : Inport  Port=3
  Fcn : Fcn  Expr=u[3]*Wp_shx1/mp_shxm*(u[1]-u[4]) + u[3]*Wp_shx2/mp_shxm*(u[2]-u[4])
  Integrator : Integrator  InitialCondition=T0_p_shx1(4)
  Mux : Mux
  Tp_shx_mix : Outport
  wires:
  Tp_shx1/1 -> Mux/1
  Tp_shx2/1 -> Mux/2
  Mux/1 -> Fcn/1
  p_flow_frac/1 -> Mux/3
  Fcn/1 -> Integrator/1
  Integrator/1 -> Tp_shx_mix/1, Mux/4

== system MSDR_v1.1/HEAT EXCHANGERS/HEAT EXCHANGER LOOP 1/SHX SEC MIXING ==
  Ts_shx1 : Inport
  Ts_shx2 : Inport  Port=2
  s_flow_frac : Inport  Port=3
  Fcn : Fcn  Expr=u[3]*Ws_shx1/ms_shxm*(u[1]-u[4]) + u[3]*Ws_shx2/ms_shxm*(u[2]-u[4])
  Integrator : Integrator  InitialCondition=T0_s_shx1(4)
  Mux : Mux
  Ts_shx_mix : Outport
  wires:
  Ts_shx1/1 -> Mux/1
  Ts_shx2/1 -> Mux/2
  Mux/1 -> Fcn/1
  s_flow_frac/1 -> Mux/3
  Fcn/1 -> Integrator/1
  Integrator/1 -> Ts_shx_mix/1, Mux/4

== system MSDR_v1.1/HEAT EXCHANGERS/HEAT EXCHANGER LOOP 1/SHX//THX PUMP ==
  1-D Lookup Table : Lookup_n-D  NumberOfTableDimensions=1  BreakpointsForDimension1=xdat  Table=ydat  InternalRulePriority=Speed  RndMeth=Simplest  InputSameDT=on
  Clock : Clock
  Fcn : Fcn  Expr=exp((1/tau_p)*u)
  Final convection flow rate : Constant  Value=therm_conv
  Scope : Scope
  Subtract : Sum  Inputs=-+
  Switch : Switch  Criteria=u2 > Threshold
  Transport Delay : TransportDelay  DelayTime=20000000  InitialOutput=1
  FLOW FRACTION : Outport
  HEAT TRANSFER FRACTION : Outport  Port=2
  wires:
  Transport Delay/1 -> 1-D Lookup Table/1, Scope/1, FLOW FRACTION/1
  Clock/1 -> Fcn/1
  Switch/1 -> Transport Delay/1
  Fcn/1 -> Subtract/1, Switch/1
  Final convection flow rate/1 -> Subtract/2, Switch/3
  Subtract/1 -> Switch/2
  1-D Lookup Table/1 -> HEAT TRANSFER FRACTION/1

== system MSDR_v1.1/HEAT EXCHANGERS/HEAT EXCHANGER LOOP 1/SHX1 HEAT TRANSFER ==
  PRIMARY FLUID INLET TEMPERATURE : Inport
  SECONDARY FLUID INLET TEMPERATURE : Inport  Port=2
  PRIMARY FLOW FRACTION : Inport  Port=3
  PRIMARY HEAT TRANSFER FRACTION : Inport  Port=4
  SECONDARY FLOW FRACTION : Inport  Port=5
  SECONDARY HEAT TRANSFER FRACTION : Inport  Port=6
  Mux : Mux  Inputs=16
      settings: DisplayOption=signals
  To Workspace : ToWorkspace  VariableName=shx1_ht  SampleTime=-1
  Tp1_shx1 : Integrator  InitialCondition=T0_p_shx1(1)
  Tp2_shx1 : Integrator  InitialCondition=T0_p_shx1(2)
  "Tp3_shx1 " : Integrator  InitialCondition=T0_p_shx1(3)
  Tp4_shx1 : Integrator  InitialCondition=T0_p_shx1(4)
  Ts1_shx1 : Integrator  InitialCondition=T0_s_shx1(1)
  Ts2_shx1 : Integrator  InitialCondition=T0_s_shx1(2)
  Ts3_shx1 : Integrator  InitialCondition=T0_s_shx1(3)
  Ts4_shx1 : Integrator  InitialCondition=T0_s_shx1(4)
  Tt1_shx1 : Integrator  InitialCondition=T0_t_shx1(1)
  Tt2_shx1 : Integrator  InitialCondition=T0_t_shx1(2)
  d(Tp1_shx1)/dt : Fcn  Expr=(u[13]*Wp_shx1/mp_shx1(1))*(u[1] - u[3]) + (u[14]*hA_p_shx1(1)/mcp_p_shx1(1))*(u[7] - u[3])
  d(Tp2_shx1)/dt : Fcn  Expr=(u[13]*Wp_shx1/mp_shx1(2))*(u[3] - u[4]) + (u[14]*hA_p_shx1(2)/mcp_p_shx1(2))*(u[7] - u[3])
  d(Tp3_shx1)/dt : Fcn  Expr=(u[13]*Wp_shx1/mp_shx1(3))*(u[4] - u[5]) + (u[14]*hA_p_shx1(3)/mcp_p_shx1(3))*(u[8] - u[5])
  d(Tp4_shx1)/dt : Fcn  Expr=(u[13]*Wp_shx1/mp_shx1(4))*(u[5] - u[6]) + (u[14]*hA_p_shx1(4)/mcp_p_shx1(4))*(u[8] - u[5])
  d(Ts1_shx1)/dt : Fcn  Expr=(u[15]*Ws_shx1/ms_shx1(1))*(u[2] - u[9]) + (u[16]*hA_s_shx1(1)/mcp_s_shx1(1))*(u[8] - u[9])
  d(Ts2_shx1)/dt : Fcn  Expr=(u[15]*Ws_shx1/ms_shx1(2))*(u[9] - u[10]) + (u[16]*hA_s_shx1(2)/mcp_s_shx1(2))*(u[8] - u[9])
  d(Ts3_shx1)/dt : Fcn  Expr=(u[15]*Ws_shx1/ms_shx1(3))*(u[10] - u[11]) + (u[16]*hA_s_shx1(3)/mcp_s_shx1(3))*(u[7] - u[11])
  d(Ts4_shx1)/dt : Fcn  Expr=(u[15]*Ws_shx1/ms_shx1(4))*(u[11] - u[12]) + (u[16]*hA_s_shx1(4)/mcp_s_shx1(4))*(u[7] - u[11])
  d(Tt1_shx1)/dt : Fcn  Expr=(u[14]*(hA_p_shx1(1) + hA_p_shx1(2))/mcp_t_shx1(1))*(u[3] - u[7]) + (u[16]*(hA_s_shx1(1) + hA_s_shx1(2))/mcp_t_shx1(1))*(u[11] - u[7])
  d(Tt2_shx1)/dt : Fcn  Expr=(u[14]*(hA_p_shx1(3) + hA_p_shx1(4))/mcp_t_shx1(2))*(u[5] - u[8]) + (u[16]*(hA_s_shx1(3) + hA_s_shx1(4))/mcp_t_shx1(2))*(u[9] - u[8])
  SHX1 TEMPERATURES : Outport
  wires:
  Ts1_shx1/1 -> Mux/9
  Ts2_shx1/1 -> Mux/10
  d(Ts2_shx1)/dt/1 -> Ts2_shx1/1
  d(Tp4_shx1)/dt/1 -> Tp4_shx1/1
  Tt1_shx1/1 -> Mux/7
  d(Tp2_shx1)/dt/1 -> Tp2_shx1/1
  Tp4_shx1/1 -> Mux/6
  d(Tt2_shx1)/dt/1 -> Tt2_shx1/1
  SECONDARY FLUID INLET TEMPERATURE/1 -> Mux/2
  Tt2_shx1/1 -> Mux/8
  Mux/1 -> To Workspace/1, SHX1 TEMPERATURES/1, d(Ts4_shx1)/dt/1, d(Ts3_shx1)/dt/1, d(Ts2_shx1)/dt/1, d(Ts1_shx1)/dt/1, d(Tt2_shx1)/dt/1, d(Tt1_shx1)/dt/1, d(Tp4_shx1)/dt/1, d(Tp3_shx1)/dt/1, d(Tp2_shx1)/dt/1, d(Tp1_shx1)/dt/1
  d(Tp1_shx1)/dt/1 -> Tp1_shx1/1
  d(Ts4_shx1)/dt/1 -> Ts4_shx1/1
  Tp1_shx1/1 -> Mux/3
  d(Ts1_shx1)/dt/1 -> Ts1_shx1/1
  d(Ts3_shx1)/dt/1 -> Ts3_shx1/1
  Ts3_shx1/1 -> Mux/11
  Ts4_shx1/1 -> Mux/12
  "Tp3_shx1 "/1 -> Mux/5
  d(Tp3_shx1)/dt/1 -> "Tp3_shx1 "/1
  Tp2_shx1/1 -> Mux/4
  d(Tt1_shx1)/dt/1 -> Tt1_shx1/1
  PRIMARY FLUID INLET TEMPERATURE/1 -> Mux/1
  PRIMARY HEAT TRANSFER FRACTION/1 -> Mux/14
  SECONDARY HEAT TRANSFER FRACTION/1 -> Mux/16
  PRIMARY FLOW FRACTION/1 -> Mux/13
  SECONDARY FLOW FRACTION/1 -> Mux/15

== system MSDR_v1.1/HEAT EXCHANGERS/HEAT EXCHANGER LOOP 1/SHX1 MATERIAL TRANSPORT ==
  SHX1 TEMPERATURES : Inport
  wires:
  SHX1 TEMPERATURES/1 -> ?

== system MSDR_v1.1/HEAT EXCHANGERS/HEAT EXCHANGER LOOP 1/SHX2 HEAT TRANSFER ==
  PRIMARY FLUID INLET TEMPERATURE : Inport
  SECONDARY FLUID INLET TEMPERATURE : Inport  Port=2
  PRIMARY FLOW FRACTION : Inport  Port=3
  PRIMARY HEAT TRANSFER FRACTION : Inport  Port=4
  SECONDARY FLOW FRACTION : Inport  Port=5
  SECONDARY HEAT TRANSFER FRACTION : Inport  Port=6
  Mux : Mux  Inputs=16
      settings: DisplayOption=signals
  To Workspace : ToWorkspace  VariableName=shx2_ht  SampleTime=-1
  Tp1_shx2 : Integrator  InitialCondition=T0_p_shx2(1)
  Tp2_shx2 : Integrator  InitialCondition=T0_p_shx2(2)
  "Tp3_shx2 " : Integrator  InitialCondition=T0_p_shx2(3)
  Tp4_shx2 : Integrator  InitialCondition=T0_p_shx2(4)
  Ts1_shx2 : Integrator  InitialCondition=T0_s_shx2(1)
  Ts2_shx2 : Integrator  InitialCondition=T0_s_shx2(2)
  Ts3_shx2 : Integrator  InitialCondition=T0_s_shx2(3)
  Ts4_shx2 : Integrator  InitialCondition=T0_s_shx2(4)
  Tt1_shx2 : Integrator  InitialCondition=T0_t_shx2(1)
  Tt2_shx2 : Integrator  InitialCondition=T0_t_shx2(2)
  d(Tp1_shx2)/dt : Fcn  Expr=(u[13]*Wp_shx2/mp_shx2(1))*(u[1] - u[3]) + (u[14]*hA_p_shx2(1)/mcp_p_shx2(1))*(u[7] - u[3])
  d(Tp2_shx2)/dt : Fcn  Expr=(u[13]*Wp_shx2/mp_shx2(2))*(u[3] - u[4]) + (u[14]*hA_p_shx2(2)/mcp_p_shx2(2))*(u[7] - u[3])
  d(Tp3_shx2)/dt : Fcn  Expr=(u[13]*Wp_shx2/mp_shx2(3))*(u[4] - u[5]) + (u[14]*hA_p_shx2(3)/mcp_p_shx2(3))*(u[8] - u[5])
  d(Tp4_shx2)/dt : Fcn  Expr=(u[13]*Wp_shx2/mp_shx2(4))*(u[5] - u[6]) + (u[14]*hA_p_shx2(4)/mcp_p_shx2(4))*(u[8] - u[5])
  d(Ts1_shx2)/dt : Fcn  Expr=(u[15]*Ws_shx2/ms_shx2(1))*(u[2] - u[9]) + (u[16]*hA_s_shx2(1)/mcp_s_shx2(1))*(u[8] - u[9])
  d(Ts2_shx2)/dt : Fcn  Expr=(u[15]*Ws_shx2/ms_shx2(2))*(u[9] - u[10]) + (u[16]*hA_s_shx2(2)/mcp_s_shx2(2))*(u[8] - u[9])
  d(Ts3_shx2)/dt : Fcn  Expr=(u[15]*Ws_shx2/ms_shx2(3))*(u[10] - u[11]) + (u[16]*hA_s_shx2(3)/mcp_s_shx2(3))*(u[7] - u[11])
  d(Ts4_shx2)/dt : Fcn  Expr=(u[15]*Ws_shx2/ms_shx2(4))*(u[11] - u[12]) + (u[16]*hA_s_shx2(4)/mcp_s_shx2(4))*(u[7] - u[11])
  d(Tt1_shx2)/dt : Fcn  Expr=(u[14]*(hA_p_shx2(1) + hA_p_shx2(2))/mcp_t_shx2(1))*(u[3] - u[7]) + (u[16]*(hA_s_shx2(1) + hA_s_shx2(2))/mcp_t_shx2(1))*(u[11] - u[7])
  d(Tt2_shx2)/dt : Fcn  Expr=(u[14]*(hA_p_shx2(3) + hA_p_shx2(4))/mcp_t_shx2(2))*(u[5] - u[8]) + (u[16]*(hA_s_shx2(3) + hA_s_shx2(4))/mcp_t_shx2(2))*(u[9] - u[8])
  SHX2 TEMPERATURES : Outport
  wires:
  Ts1_shx2/1 -> Mux/9
  Ts2_shx2/1 -> Mux/10
  d(Ts2_shx2)/dt/1 -> Ts2_shx2/1
  d(Tp4_shx2)/dt/1 -> Tp4_shx2/1
  Tt1_shx2/1 -> Mux/7
  d(Tp2_shx2)/dt/1 -> Tp2_shx2/1
  Tp4_shx2/1 -> Mux/6
  d(Tt2_shx2)/dt/1 -> Tt2_shx2/1
  SECONDARY FLUID INLET TEMPERATURE/1 -> Mux/2
  Tt2_shx2/1 -> Mux/8
  Mux/1 -> To Workspace/1, SHX2 TEMPERATURES/1, d(Ts4_shx2)/dt/1, d(Ts3_shx2)/dt/1, d(Ts2_shx2)/dt/1, d(Ts1_shx2)/dt/1, d(Tt2_shx2)/dt/1, d(Tt1_shx2)/dt/1, d(Tp4_shx2)/dt/1, d(Tp3_shx2)/dt/1, d(Tp2_shx2)/dt/1, d(Tp1_shx2)/dt/1
  d(Tp1_shx2)/dt/1 -> Tp1_shx2/1
  d(Ts4_shx2)/dt/1 -> Ts4_shx2/1
  Tp1_shx2/1 -> Mux/3
  d(Ts1_shx2)/dt/1 -> Ts1_shx2/1
  d(Ts3_shx2)/dt/1 -> Ts3_shx2/1
  Ts3_shx2/1 -> Mux/11
  Ts4_shx2/1 -> Mux/12
  "Tp3_shx2 "/1 -> Mux/5
  d(Tp3_shx2)/dt/1 -> "Tp3_shx2 "/1
  Tp2_shx2/1 -> Mux/4
  d(Tt1_shx2)/dt/1 -> Tt1_shx2/1
  PRIMARY FLUID INLET TEMPERATURE/1 -> Mux/1
  PRIMARY HEAT TRANSFER FRACTION/1 -> Mux/14
  SECONDARY FLOW FRACTION/1 -> Mux/15
  SECONDARY HEAT TRANSFER FRACTION/1 -> Mux/16
  PRIMARY FLOW FRACTION/1 -> Mux/13

== system MSDR_v1.1/HEAT EXCHANGERS/HEAT EXCHANGER LOOP 1/SHX2 MATERIAL TRANSPORT ==
  SHX2 TEMPERATURES : Inport
  wires:
  SHX2 TEMPERATURES/1 -> ?

== system MSDR_v1.1/HEAT EXCHANGERS/HEAT EXCHANGER LOOP 2/BOILER & REHEATER ==
  Coolant Inlet Temp : Inport
  Power Demand (Frac) : Inport  Port=2
  Fcn : Fcn  Commented=on  Expr=u[1] - u[2]*250/((Ws_shx1 + Ws_shx2)*Cp_s_shx)
  Integrator : Integrator  InitialCondition=400
  Mux : Mux  Inputs=3
      settings: DisplayOption=signals
  To Workspace : ToWorkspace  VariableName=msdr_br_mux2  SampleTime=-1
  ddt_t_b = 1/tau_b*(t_bin-t_b)-p_b/mb_cpb : Fcn  Expr=W_sb*(u(1)-u(3))/m_sb - u(2)/mb_cpb
  Coolant Exit Temp : Outport
  wires:
  Integrator/1 -> Coolant Exit Temp/1, Mux/3
  Mux/1 -> ddt_t_b = 1/tau_b*(t_bin-t_b)-p_b/mb_cpb/1, To Workspace/1
  Power Demand (Frac)/1 -> Mux/2
  Coolant Inlet Temp/1 -> Mux/1
  ddt_t_b = 1/tau_b*(t_bin-t_b)-p_b/mb_cpb/1 -> Integrator/1

== system MSDR_v1.1/HEAT EXCHANGERS/HEAT EXCHANGER LOOP 2/Fractional Power Demand (fractional) ==
  Add : Sum
  Constant : Constant
  Saturation : Saturate  UpperLimit=1  LowerLimit=0.2
  Saturation1 : Saturate  UpperLimit=.8  LowerLimit=0
  Slider : Subsystem  DialogController=hmiCreateDDGDialog  IsWebBlock=on  mask(MWDashboardBlock){webBlockId=d640d4ad-cb91-4634-9ac2-9a3bc57b8e2e, webBlockType=slider, ShowInLibBrowser=on, ShowInitialText=on, HMISrcModelName=OTSG_v1_1}
      mask prompts: webBlockId "WebBlock Id"; webBlockType "WebBlock Type"; HMISrcModelName "Source Model"
      mask help: SimulinkHMI:dialogs:SliderDialogDesc
      mask Help: helpview([docroot '/mapfiles/simulink.map'], 'hmi_slider')
      mask Display:
      | if strcmp(get_param(bdroot(gcb),'BlockDiagramType'), 'library')
      |     image([(matlabroot) '/toolbox/simulink/hmi/icons/Slider.png']);
      | end
  down 1%/min : simulink/Sources/Ramp  slope=-0.01/60  start=2500  InitialOutput=1
  up 1%/min1 : simulink/Sources/Ramp  slope=0.01/60  start=2500+3600+5000  InitialOutput=0
  Power Demand(frac) : Outport
  wires:
  down 1%/min/1 -> Saturation/1
  Saturation/1 -> Add/1
  up 1%/min1/1 -> Saturation1/1
  Saturation1/1 -> Add/2
  Constant/1 -> Power Demand(frac)/1

== system MSDR_v1.1/HEAT EXCHANGERS/HEAT EXCHANGER LOOP 2/PHX PRIM MIXING ==
  Tp_phx3 : Inport
  Tp_phx4 : Inport  Port=2
  p_flow_frac : Inport  Port=3
  Fcn : Fcn  Expr=u[3]*Wp_phx3/mp_phxm*(u[1]-u[4]) + u[3]*Wp_phx4/mp_phxm*(u[2]-u[4])
  Integrator : Integrator  InitialCondition=Tf_in
  Mux : Mux
  Tp_phx_mix : Outport
  wires:
  Tp_phx3/1 -> Mux/1
  Tp_phx4/1 -> Mux/2
  Mux/1 -> Fcn/1
  p_flow_frac/1 -> Mux/3
  Fcn/1 -> Integrator/1
  Integrator/1 -> Tp_phx_mix/1, Mux/4

== system MSDR_v1.1/HEAT EXCHANGERS/HEAT EXCHANGER LOOP 2/PHX SEC MIXING ==
  Ts_phx3 : Inport
  Ts_phx4 : Inport  Port=2
  s_flow_frac : Inport  Port=3
  Fcn : Fcn  Expr=u[3]*Ws_phx3/ms_phxm*(u[1]-u[4]) + u[3]*Ws_phx4/ms_phxm*(u[2]-u[4])
  Integrator : Integrator  InitialCondition=T0_s_phx1(4)
  Mux : Mux
  Ts_phx_mix : Outport
  wires:
  Ts_phx3/1 -> Mux/1
  Ts_phx4/1 -> Mux/2
  Mux/1 -> Fcn/1
  s_flow_frac/1 -> Mux/3
  Fcn/1 -> Integrator/1
  Integrator/1 -> Ts_phx_mix/1, Mux/4

== system MSDR_v1.1/HEAT EXCHANGERS/HEAT EXCHANGER LOOP 2/PHX//SHX PUMP ==
  1-D Lookup Table : Lookup_n-D  NumberOfTableDimensions=1  BreakpointsForDimension1=xdat  Table=ydat  InternalRulePriority=Speed  RndMeth=Simplest  InputSameDT=on
  Clock : Clock
  Fcn : Fcn  Expr=exp((1/tau_p)*u)
  Final convection flow rate : Constant  Value=therm_conv
  Scope : Scope
  Subtract : Sum  Inputs=-+
  Switch : Switch  Criteria=u2 > Threshold
  Transport Delay : TransportDelay  DelayTime=60000000  InitialOutput=1
  FLOW FRACTION : Outport
  HEAT TRANSFER FRACTION : Outport  Port=2
  wires:
  Transport Delay/1 -> 1-D Lookup Table/1, Scope/1, FLOW FRACTION/1
  Clock/1 -> Fcn/1
  Switch/1 -> Transport Delay/1
  Fcn/1 -> Subtract/1, Switch/1
  Final convection flow rate/1 -> Subtract/2, Switch/3
  Subtract/1 -> Switch/2
  1-D Lookup Table/1 -> HEAT TRANSFER FRACTION/1

== system MSDR_v1.1/HEAT EXCHANGERS/HEAT EXCHANGER LOOP 2/PHX3 HEAT TRANSFER ==
  PRIMARY FLUID INLET TEMPERATURE : Inport
  SECONDARY FLUID INLET TEMPERATURE : Inport  Port=2
  PRIMARY FLOW FRACTION : Inport  Port=3
  PRIMARY HEAT TRANSFER FRACTION : Inport  Port=4
  SECONDARY FLOW FRACTION : Inport  Port=5
  SECONDARY HEAT TRANSFER FRACTION : Inport  Port=6
  Mux : Mux  Inputs=16
      settings: DisplayOption=signals
  To Workspace : ToWorkspace  VariableName=phx3_ht  SampleTime=-1
  Tp1_phx3 : Integrator  InitialCondition=T0_p_phx3(1)
  Tp2_phx3 : Integrator  InitialCondition=T0_p_phx3(2)
  "Tp3_phx3 " : Integrator  InitialCondition=T0_p_phx3(3)
  Tp4_phx3 : Integrator  InitialCondition=T0_p_phx3(4)
  Ts1_phx3 : Integrator  InitialCondition=T0_s_phx3(1)
  Ts2_phx3 : Integrator  InitialCondition=T0_s_phx3(2)
  Ts3_phx3 : Integrator  InitialCondition=T0_s_phx3(3)
  Ts4_phx3 : Integrator  InitialCondition=T0_s_phx3(4)
  Tt1_phx3 : Integrator  InitialCondition=T0_t_phx3(1)
  Tt2_phx3 : Integrator  InitialCondition=T0_t_phx3(2)
  d(Tp1_phx3)/dt : Fcn  Expr=(u[13]*Wp_phx3/mp_phx3(1))*(u[1] - u[3]) + (u[14]*hA_p_phx3(1)/mcp_p_phx3(1))*(u[7] - u[3])
  d(Tp2_phx3)/dt : Fcn  Expr=(u[13]*Wp_phx3/mp_phx3(2))*(u[3] - u[4]) + (u[14]*hA_p_phx3(2)/mcp_p_phx3(2))*(u[7] - u[3])
  d(Tp3_phx3)/dt : Fcn  Expr=(u[13]*Wp_phx3/mp_phx3(3))*(u[4] - u[5]) + (u[14]*hA_p_phx3(3)/mcp_p_phx3(3))*(u[8] - u[5])
  d(Tp4_phx3)/dt : Fcn  Expr=(u[13]*Wp_phx3/mp_phx3(4))*(u[5] - u[6]) + (u[14]*hA_p_phx3(4)/mcp_p_phx3(4))*(u[8] - u[5])
  d(Ts1_phx3)/dt : Fcn  Expr=(u[15]*Ws_phx3/ms_phx3(1))*(u[2] - u[9]) + (u[16]*hA_s_phx3(1)/mcp_s_phx3(1))*(u[8] - u[9])
  d(Ts2_phx3)/dt : Fcn  Expr=(u[15]*Ws_phx3/ms_phx3(2))*(u[9] - u[10]) + (u[16]*hA_s_phx3(2)/mcp_s_phx3(2))*(u[8] - u[9])
  d(Ts3_phx3)/dt : Fcn  Expr=(u[15]*Ws_phx3/ms_phx3(3))*(u[10] - u[11]) + (u[16]*hA_s_phx3(3)/mcp_s_phx3(3))*(u[7] - u[11])
  d(Ts4_phx3)/dt : Fcn  Expr=(u[15]*Ws_phx3/ms_phx3(4))*(u[11] - u[12]) + (u[16]*hA_s_phx3(4)/mcp_s_phx3(4))*(u[7] - u[11])
  d(Tt1_phx3)/dt : Fcn  Expr=(u[14]*(hA_p_phx3(1) + hA_p_phx3(2))/mcp_t_phx3(1))*(u[3] - u[7]) + (u[16]*(hA_s_phx3(1) + hA_s_phx3(2))/mcp_t_phx3(1))*(u[11] - u[7])
  d(Tt2_phx3)/dt : Fcn  Expr=(u[14]*(hA_p_phx3(3) + hA_p_phx3(4))/mcp_t_phx3(2))*(u[5] - u[8]) + (u[16]*(hA_s_phx3(3) + hA_s_phx3(4))/mcp_t_phx3(2))*(u[9] - u[8])
  PHX3 TEMPERATURES : Outport
  wires:
  Ts1_phx3/1 -> Mux/9
  Ts2_phx3/1 -> Mux/10
  d(Ts2_phx3)/dt/1 -> Ts2_phx3/1
  d(Tp4_phx3)/dt/1 -> Tp4_phx3/1
  Tt1_phx3/1 -> Mux/7
  d(Tp2_phx3)/dt/1 -> Tp2_phx3/1
  Tp4_phx3/1 -> Mux/6
  d(Tt2_phx3)/dt/1 -> Tt2_phx3/1
  SECONDARY FLUID INLET TEMPERATURE/1 -> Mux/2
  Tt2_phx3/1 -> Mux/8
  Mux/1 -> To Workspace/1, PHX3 TEMPERATURES/1, d(Ts4_phx3)/dt/1, d(Ts3_phx3)/dt/1, d(Ts1_phx3)/dt/1, d(Tt2_phx3)/dt/1, d(Tt1_phx3)/dt/1, d(Tp4_phx3)/dt/1, d(Tp3_phx3)/dt/1, d(Tp2_phx3)/dt/1, d(Tp1_phx3)/dt/1, d(Ts2_phx3)/dt/1
  d(Tp1_phx3)/dt/1 -> Tp1_phx3/1
  d(Ts4_phx3)/dt/1 -> Ts4_phx3/1
  Tp1_phx3/1 -> Mux/3
  d(Ts1_phx3)/dt/1 -> Ts1_phx3/1
  d(Ts3_phx3)/dt/1 -> Ts3_phx3/1
  Ts3_phx3/1 -> Mux/11
  Ts4_phx3/1 -> Mux/12
  "Tp3_phx3 "/1 -> Mux/5
  d(Tp3_phx3)/dt/1 -> "Tp3_phx3 "/1
  Tp2_phx3/1 -> Mux/4
  d(Tt1_phx3)/dt/1 -> Tt1_phx3/1
  PRIMARY FLUID INLET TEMPERATURE/1 -> Mux/1
  PRIMARY FLOW FRACTION/1 -> Mux/13
  PRIMARY HEAT TRANSFER FRACTION/1 -> Mux/14
  SECONDARY FLOW FRACTION/1 -> Mux/15
  SECONDARY HEAT TRANSFER FRACTION/1 -> Mux/16

== system MSDR_v1.1/HEAT EXCHANGERS/HEAT EXCHANGER LOOP 2/PHX3 MATERIAL TRANSPORT ==
  PHX3 TEMPERATURES : Inport
  wires:
  PHX3 TEMPERATURES/1 -> ?
